simulink model "EVSR24"  (R2022b)
settings: Solver=VariableStepAuto  StartTime=0.0  StopTime=10.0  RelTol=1e-3
settings Model: Creator=serga  LastModifiedBy=serga

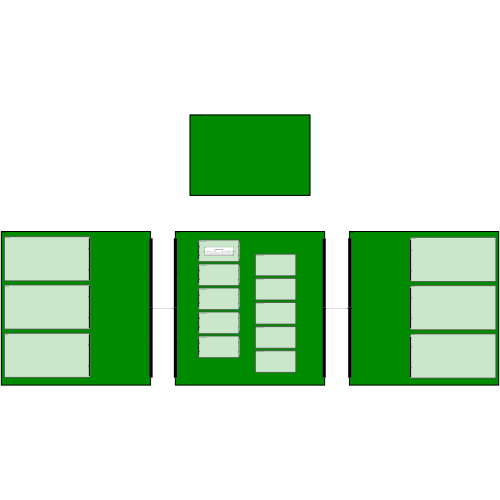
[thumbnail: Simulink's stored preview of the top-level diagram]
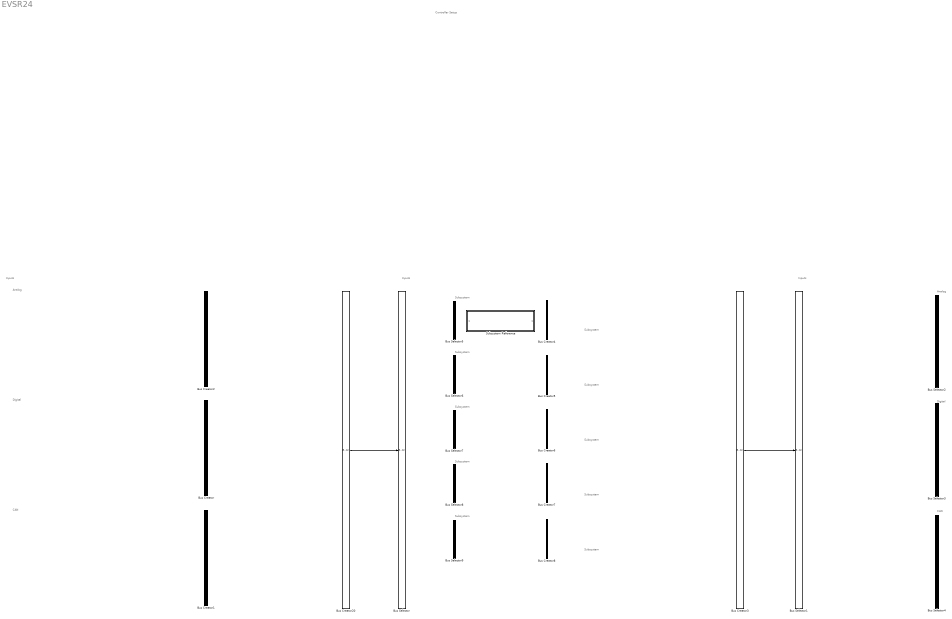
== system EVSR24 ==
  note: Controller Setup
  note: Inputs
  note: Analog
  note: Digital
  note: CAN
  note: Inputs
  note: Inputs
  note: Digital
  note: CAN
  note: Analog
  note: Subsystem
  note: Subsystem
  note: Subsystem
  note: Subsystem
  note: Subsystem
  note: Subsystem
  note: Subsystem
  note: Subsystem
  note: Subsystem
  note: Subsystem
  Bus Creator{,1..8,20} (10 alike) : BusCreator  Inputs=2
  Bus Selector{,1..9} (10 alike) : BusSelector  OutputSignals=signal1,signal2
  Subsystem Reference : Subsystem  ReferencedSubsystem=motorcontroller
  wires:
  Bus Creator20/1 -> Bus Selector/1
  Bus Creator3/1 -> Bus Selector1/1
